simulink model "j51"  (R2015b)
settings: Solver=VariableStepAuto  StartTime=-10  StopTime=10.0  RelTol=1e-3
libraries: simulink x1
settings Model: Creator=Pouya  LastModifiedBy=Pouya

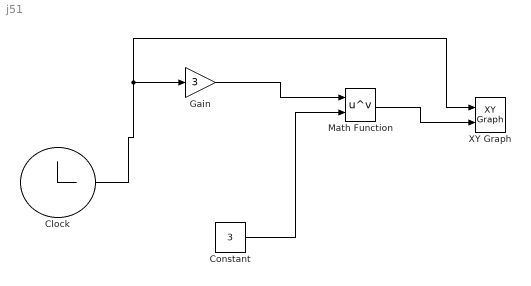
== system j51 ==
  Clock : Clock
  Constant : Constant  Value=3
  Gain : Gain  Gain=3
  Math Function : Math  Operator=pow  SaturateOnIntegerOverflow=on
  XY Graph : simulink/Sinks/XY Graph  xmin=-2  xmax=2  ymin=-100  ymax=100  st=-1
  wires:
  Math Function/1 -> XY Graph/2
  Clock/1 -> XY Graph/1, Gain/1
  Gain/1 -> Math Function/1
  Constant/1 -> Math Function/2
